simulink model "Model1"  (R2017a)
settings: Solver=ode23  StartTime=0.0  StopTime=10.0  RelTol=1e-8
values from neighbouring files (symbols this model uses):
  param = evalin('base','param')    [getSaveInfo.m]    (also in loadBackUp.m)
  u1 = 5    [Debug1.m]    (also in Model1Debug.m = 1)
  u2 = 0    [Debug1.m]    (also in Model1Debug.m)
  u3 = 0    [Debug1.m]    (also in Model1Debug.m)
  u4 = 0    [Debug1.m]    (also in Model1Debug.m = 3.25)
  u5 = 0    [Debug1.m]    (also in Model1Debug.m)
(part 3 of 3)

== matlab function Model1/RTR+(2,0)/MATLAB Function1 ==
  data: Q output; QT output; q input; Qdet output
function [Q,QT,Qdet]  = fcn(q)

c1=cos(q(1));
c2=cos(q(2));
c3=cos(q(3));

s1=sin(q(1));
s2=sin(q(2));
s3=sin(q(3));
Q=[0.247589583333333333E3+(100/9).*(4+(18/5).*c1+(6/5).*c3+(4/5).* ...
  c1.*c3+(4/15).*c3.^2)+(-20/3).*(9+2.*c3).*s1, ...
  0.604104166666666667E2+(-100/9).*(4+(18/5).*c1+(6/5).*c3+(4/5).* ...
  c1.*c3+(4/15).*c3.^2),(10/3).*((12/5)+(9/5).*c1+(2/5).*c1.*c3+( ...
  4/15).*c3.^2)+(-1).*(9+2.*c3).*s1,0,(-2).*c1.*s3+(-4/3).*s1.*s3; ...
  0.604104166666666667E2+(-100/9).*(4+(18/5).*c1+(6/5).*c3+(4/5).* ...
  c1.*c3+(4/15).*c3.^2),0.247589583333333333E3+(100/9).*(4+(18/5).* ...
  c1+(6/5).*c3+(4/5).*c1.*c3+(4/15).*c3.^2)+(20/3).*(9+2.*c3).*s1,( ...
  -10/3).*((12/5)+(9/5).*c1+(2/5).*c1.*c3+(4/15).*c3.^2)+(-1).*(9+ ...
  2.*c3).*s1,0,(-2).*c1.*s3+(4/3).*s1.*s3;(10/3).*((12/5)+(9/5).*c1+ ...
  (2/5).*c1.*c3+(4/15).*c3.^2)+(-1).*(9+2.*c3).*s1,(-10/3).*((12/5)+ ...
  (9/5).*c1+(2/5).*c1.*c3+(4/15).*c3.^2)+(-1).*(9+2.*c3).*s1,(12/5)+ ...
  (6/5).*c3+(4/15).*c3.^2,0,0;0,0,0,40,2.*c3;(-2).*c1.*s3+(-4/3).* ...
  s1.*s3,(-2).*c1.*s3+(4/3).*s1.*s3,0,2.*c3,(4/15)];
Qinv=inv(Q);
QT=transpose(Q);
Qdet=det(Q);

== matlab function Model1/RTR+(2,0)/MATLAB Function2 ==
  data: C output; q input; qp input; qap input; CT output
function [C,CT]= fcn(q,qp,qap)

c1=cos(q(1));
c2=cos(q(2));
c3=cos(q(3));

s1=sin(q(1));
s2=sin(q(2));
s3=sin(q(3));

C=[(10/3).*c1.*((-9)+(-2).*c3).*qp(6)+(20/3).*qp(8).*s1.*s3+(100/9).*( ...
  qp(6).*((-9/5).*s1+(-2/5).*c3.*s1)+(-1).*qp(8).*((3/5).*s3+(2/5).*c1.* ...
  s3+(4/15).*c3.*s3)),(20/3).*(8+c1.*(9+2.*c3)).*qp(3)+(-10/3).*c1.*(( ...
  -9)+(-2).*c3).*qp(6)+(-20/3).*qp(8).*s1.*s3+(-100/9).*(qp(6).*((-9/5).* ...
  s1+(-2/5).*c3.*s1)+(-1).*qp(8).*((3/5).*s3+(2/5).*c1.*s3+(4/15).* ...
  c3.*s3)),(-1).*c1.*(9+2.*c3).*(qp(3)+qp(6))+2.*qp(8).*s1.*s3+(10/3).*(( ...
  qp(3)+qp(6)).*((-9/5).*s1+(-2/5).*c3.*s1)+(-1).*qp(8).*((2/5).*c1.*s3+( ...
  4/15).*c3.*s3)),0,(-2).*c1.*c3.*qp(8)+2.*(qp(3)+qp(6)).*s1.*s3+(10/3).*( ...
  (-2/5).*c3.*qp(8).*s1+(-1).*qp(6).*((2/5).*c1.*s3+(4/15).*c3.*s3)+(-1) ...
  .*qp(3).*((3/5).*s3+(2/5).*c1.*s3+(4/15).*c3.*s3));(-20/3).*(8+c1.*( ...
  9+2.*c3)).*qp(3)+(10/3).*c1.*((-9)+(-2).*c3).*qp(6)+(20/3).*qp(8).*s1.* ...
  s3+(-100/9).*(qp(6).*((-9/5).*s1+(-2/5).*c3.*s1)+(-1).*qp(8).*((3/5).* ...
  s3+(2/5).*c1.*s3+(4/15).*c3.*s3)),(-10/3).*c1.*((-9)+(-2).*c3).* ...
  qp(6)+(-20/3).*qp(8).*s1.*s3+(100/9).*(qp(6).*((-9/5).*s1+(-2/5).*c3.* ...
  s1)+(-1).*qp(8).*((3/5).*s3+(2/5).*c1.*s3+(4/15).*c3.*s3)),(-1).* ...
  c1.*(9+2.*c3).*(qp(3)+qp(6))+2.*qp(8).*s1.*s3+(-10/3).*((qp(3)+qp(6)).*(( ...
  -9/5).*s1+(-2/5).*c3.*s1)+(-1).*qp(8).*((2/5).*c1.*s3+(4/15).*c3.* ...
  s3)),0,(-2).*c1.*c3.*qp(8)+2.*(qp(3)+qp(6)).*s1.*s3+(-10/3).*((-2/5).* ...
  c3.*qp(8).*s1+(-1).*qp(6).*((2/5).*c1.*s3+(4/15).*c3.*s3)+(-1).*qp(3).*( ...
  (3/5).*s3+(2/5).*c1.*s3+(4/15).*c3.*s3));(10/3).*(qp(3).*((9/5).*s1+ ...
  (2/5).*c3.*s1)+(-4/75).*c3.*qp(8).*s3),(-10/3).*(qp(3).*((9/5).*s1+( ...
  2/5).*c3.*s1)+(-4/75).*c3.*qp(8).*s3),qp(8).*((-3/5).*s3+(-4/15).*c3.* ...
  s3),0,(-4/15).*c3.*qp(3).*s3+qp(6).*((-3/5).*s3+(-4/15).*c3.*s3);0,0, ...
  0,0,(-2).*qp(8).*s3;(10/3).*((4/75).*c3.*qp(6).*s3+qp(3).*((3/5).*s3+( ...
  2/5).*c1.*s3+(4/15).*c3.*s3)),(-10/3).*((4/75).*c3.*qp(6).*s3+qp(3).*( ...
  (3/5).*s3+(2/5).*c1.*s3+(4/15).*c3.*s3)),(4/15).*c3.*qp(3).*s3+(-1) ...
  .*qp(6).*((-3/5).*s3+(-4/15).*c3.*s3),0,0];
CT=C';

== matlab function Model1/RTR+(2,0)/MATLAB Function3 ==
  data: D output; q input; qp input; qap input
function D = fcn(q,qp,qap)

c1=cos(q(1));
c2=cos(q(2));
c3=cos(q(3));

s1=sin(q(1));
s2=sin(q(2));
s3=sin(q(3));

D=[0;0;0;0.392400000000000000E3;0.196200000000000000E2.*c3];
